simulink model "pid_autotuning_control"  (Simulink 5.0)
settings: Solver=FixedStepDiscrete  StartTime=0.0  StopTime=500.0  FixedStep=0.1  RelTol=1e-3
libraries: mathlib x5, genlib x2, execlib x1, reglib x1, arclib x1
settings Model: LastModifiedBy=david  ExtModeTrigMode=oneshot  ExtModeArmWhenConnect=off  LimitDataPoints=off  BooleanDataType=off

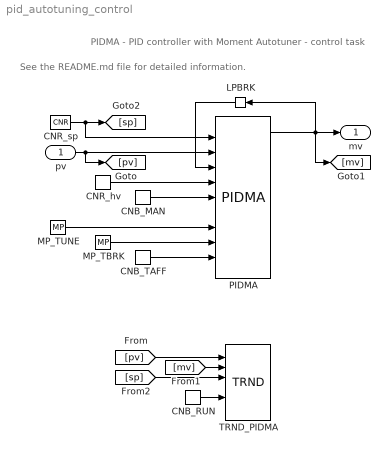
== system pid_autotuning_control ==
  note: See the README.md file for detailed information.
  note: PIDMA - PID controller with Moment Autotuner - control task
  pv : Inport  Port=1
  CNB_MAN : mathlib/CNB  YCN=on
  CNB_RUN : mathlib/CNB  YCN=on
  CNB_TAFF : mathlib/CNB  YCN=on
  CNR_hv : mathlib/CNR  ycn=0
  CNR_sp : mathlib/CNR  ycn=0
  LPBRK : execlib/LPBRK  Orientation=left
  MP_TBRK : genlib/MP  pwidth=1  BSTATE=off  RPTF=off
  MP_TUNE : genlib/MP  pwidth=1  BSTATE=off  RPTF=off
  PIDMA : reglib/PIDMA  irtype=7: PID  RACT=off  k=1  ti=5.5  td=0  nd=4  b=1  c=0  tt=1  hilim=1  lolim=-1  dz=0  icotype=1: Analog  ittype=7: PID  iainf=1: Static process  DGC=off  tdg=1  tn=2  amp=0.2  dy=0.1  ispeed=2: Normal (middle fast) CL  ipid=1: Parallel form
  TRND_PIDMA : arclib/TRND  n=3  l=1000  btype=8  ptype1=1: Store  ptype2=1: Store  ptype3=1: Store  ptype4=1: Store  pfac=1  afac=0  arc=0  id=1  Title=Trend Title  timesrc=1
  mv : Outport  Port=1
  wires:
  CNB_MAN/1 -> PIDMA/6
  CNB_RUN/1 -> TRND_PIDMA/5
  CNB_TAFF/1 -> PIDMA/10
  CNR_hv/1 -> PIDMA/5
  CNR_sp/1 -> [sp], PIDMA/2
  [pv] -> TRND_PIDMA/1
  [mv] -> TRND_PIDMA/2
  [sp] -> TRND_PIDMA/3
  LPBRK/1 -> PIDMA/4
  MP_TBRK/1 -> PIDMA/9
  MP_TUNE/1 -> PIDMA/8
  PIDMA/1 -> [mv], LPBRK/1, mv/1
  pv/1 -> [pv], PIDMA/3
